simulink model "VACModel"  (Simulink 8.3)
settings: Solver=ode1  SolverMode=MultiTasking  StartTime=0.0  StopTime=24  FixedStep=Ts_base  MaxStep=Ts_base  MinStep=1e-6  RelTol=1e-6
PreLoadFcn:
  | initModel
StopFcn:
  | overview
undefined symbols (not defined in the file): automatic, controller_sampling_frequency, Fixed, gcr, MVs, PI, signal, transmitter_deadtime, transmitter_sampling_frequency, Ts_save, y_ss
libraries: VAlib x96
(part 15 of 18)

== system VACModel/VA Plant/xmeas atk block/xmeas3 attack controller/Attack Type Controller ==
  note: 1) Only subsystems can be added as variant choices at this level
      | 2) Blocks cannot be connected at this level as connectivity is
      | automatically determined at simulation, based on the active variant
  normal : Inport
  faked : Inport  Port=2
  interval forward controller : Subsystem  VariantControl=interval_forward_controller
      mask Display:
      | disp('IFC')
      | port_label('input', 1, 'normal in')
      | port_label('input', 2, 'faked in')
      | port_label('output', 1, 'out')
  normal forward controller : Subsystem  VariantControl=normal_forward_controller
      mask Display:
      | disp('NFC')
      | port_label('input', 1, 'normal in')
      | port_label('input', 2, 'faked in')
      | port_label('output', 1, 'out')
  periodical forward controller : Subsystem  VariantControl=periodical_forward_controller
      mask Display:
      | disp('PFC')
      | port_label('input', 1, 'normal in')
      | port_label('input', 2, 'faked in')
      | port_label('output', 1, 'out')
  step forward controller : Subsystem  VariantControl=step_forward_controller
      mask Display:
      | disp('SFC')
      | port_label('input', 1, 'normal in')
      | port_label('input', 2, 'faked in')
      | port_label('output', 1, 'out')
  output : Outport

== system VACModel/VA Plant/xmeas atk block/xmeas30 attack controller/Attack Type Controller ==
  note: 1) Only subsystems can be added as variant choices at this level
      | 2) Blocks cannot be connected at this level as connectivity is
      | automatically determined at simulation, based on the active variant
  normal : Inport
  faked : Inport  Port=2
  interval forward controller : Subsystem  VariantControl=interval_forward_controller
      mask Display:
      | disp('IFC')
      | port_label('input', 1, 'normal in')
      | port_label('input', 2, 'faked in')
      | port_label('output', 1, 'out')
  normal forward controller : Subsystem  VariantControl=normal_forward_controller
      mask Display:
      | disp('NFC')
      | port_label('input', 1, 'normal in')
      | port_label('input', 2, 'faked in')
      | port_label('output', 1, 'out')
  periodical forward controller : Subsystem  VariantControl=periodical_forward_controller
      mask Display:
      | disp('PFC')
      | port_label('input', 1, 'normal in')
      | port_label('input', 2, 'faked in')
      | port_label('output', 1, 'out')
  step forward controller : Subsystem  VariantControl=step_forward_controller
      mask Display:
      | disp('SFC')
      | port_label('input', 1, 'normal in')
      | port_label('input', 2, 'faked in')
      | port_label('output', 1, 'out')
  output : Outport

== system VACModel/VA Plant/xmeas atk block/xmeas31 attack controller/Attack Type Controller ==
  note: 1) Only subsystems can be added as variant choices at this level
      | 2) Blocks cannot be connected at this level as connectivity is
      | automatically determined at simulation, based on the active variant
  normal : Inport
  faked : Inport  Port=2
  interval forward controller : Subsystem  VariantControl=interval_forward_controller
      mask Display:
      | disp('IFC')
      | port_label('input', 1, 'normal in')
      | port_label('input', 2, 'faked in')
      | port_label('output', 1, 'out')
  normal forward controller : Subsystem  VariantControl=normal_forward_controller
      mask Display:
      | disp('NFC')
      | port_label('input', 1, 'normal in')
      | port_label('input', 2, 'faked in')
      | port_label('output', 1, 'out')
  periodical forward controller : Subsystem  VariantControl=periodical_forward_controller
      mask Display:
      | disp('PFC')
      | port_label('input', 1, 'normal in')
      | port_label('input', 2, 'faked in')
      | port_label('output', 1, 'out')
  step forward controller : Subsystem  VariantControl=step_forward_controller
      mask Display:
      | disp('SFC')
      | port_label('input', 1, 'normal in')
      | port_label('input', 2, 'faked in')
      | port_label('output', 1, 'out')
  output : Outport

== system VACModel/VA Plant/xmeas atk block/xmeas32 attack controller/Attack Type Controller ==
  note: 1) Only subsystems can be added as variant choices at this level
      | 2) Blocks cannot be connected at this level as connectivity is
      | automatically determined at simulation, based on the active variant
  normal : Inport
  faked : Inport  Port=2
  interval forward controller : Subsystem  VariantControl=interval_forward_controller
      mask Display:
      | disp('IFC')
      | port_label('input', 1, 'normal in')
      | port_label('input', 2, 'faked in')
      | port_label('output', 1, 'out')
  normal forward controller : Subsystem  VariantControl=normal_forward_controller
      mask Display:
      | disp('NFC')
      | port_label('input', 1, 'normal in')
      | port_label('input', 2, 'faked in')
      | port_label('output', 1, 'out')
  periodical forward controller : Subsystem  VariantControl=periodical_forward_controller
      mask Display:
      | disp('PFC')
      | port_label('input', 1, 'normal in')
      | port_label('input', 2, 'faked in')
      | port_label('output', 1, 'out')
  step forward controller : Subsystem  VariantControl=step_forward_controller
      mask Display:
      | disp('SFC')
      | port_label('input', 1, 'normal in')
      | port_label('input', 2, 'faked in')
      | port_label('output', 1, 'out')
  output : Outport

== system VACModel/VA Plant/xmeas atk block/xmeas33 attack controller/Attack Type Controller ==
  note: 1) Only subsystems can be added as variant choices at this level
      | 2) Blocks cannot be connected at this level as connectivity is
      | automatically determined at simulation, based on the active variant
  normal : Inport
  faked : Inport  Port=2
  interval forward controller : Subsystem  VariantControl=interval_forward_controller
      mask Display:
      | disp('IFC')
      | port_label('input', 1, 'normal in')
      | port_label('input', 2, 'faked in')
      | port_label('output', 1, 'out')
  normal forward controller : Subsystem  VariantControl=normal_forward_controller
      mask Display:
      | disp('NFC')
      | port_label('input', 1, 'normal in')
      | port_label('input', 2, 'faked in')
      | port_label('output', 1, 'out')
  periodical forward controller : Subsystem  VariantControl=periodical_forward_controller
      mask Display:
      | disp('PFC')
      | port_label('input', 1, 'normal in')
      | port_label('input', 2, 'faked in')
      | port_label('output', 1, 'out')
  step forward controller : Subsystem  VariantControl=step_forward_controller
      mask Display:
      | disp('SFC')
      | port_label('input', 1, 'normal in')
      | port_label('input', 2, 'faked in')
      | port_label('output', 1, 'out')
  output : Outport

== system VACModel/VA Plant/xmeas atk block/xmeas34 attack controller/Attack Type Controller ==
  note: 1) Only subsystems can be added as variant choices at this level
      | 2) Blocks cannot be connected at this level as connectivity is
      | automatically determined at simulation, based on the active variant
  normal : Inport
  faked : Inport  Port=2
  interval forward controller : Subsystem  VariantControl=interval_forward_controller
      mask Display:
      | disp('IFC')
      | port_label('input', 1, 'normal in')
      | port_label('input', 2, 'faked in')
      | port_label('output', 1, 'out')
  normal forward controller : Subsystem  VariantControl=normal_forward_controller
      mask Display:
      | disp('NFC')
      | port_label('input', 1, 'normal in')
      | port_label('input', 2, 'faked in')
      | port_label('output', 1, 'out')
  periodical forward controller : Subsystem  VariantControl=periodical_forward_controller
      mask Display:
      | disp('PFC')
      | port_label('input', 1, 'normal in')
      | port_label('input', 2, 'faked in')
      | port_label('output', 1, 'out')
  step forward controller : Subsystem  VariantControl=step_forward_controller
      mask Display:
      | disp('SFC')
      | port_label('input', 1, 'normal in')
      | port_label('input', 2, 'faked in')
      | port_label('output', 1, 'out')
  output : Outport

== system VACModel/VA Plant/xmeas atk block/xmeas35 attack controller/Attack Type Controller ==
  note: 1) Only subsystems can be added as variant choices at this level
      | 2) Blocks cannot be connected at this level as connectivity is
      | automatically determined at simulation, based on the active variant
  normal : Inport
  faked : Inport  Port=2
  interval forward controller : Subsystem  VariantControl=interval_forward_controller
      mask Display:
      | disp('IFC')
      | port_label('input', 1, 'normal in')
      | port_label('input', 2, 'faked in')
      | port_label('output', 1, 'out')
  normal forward controller : Subsystem  VariantControl=normal_forward_controller
      mask Display:
      | disp('NFC')
      | port_label('input', 1, 'normal in')
      | port_label('input', 2, 'faked in')
      | port_label('output', 1, 'out')
  periodical forward controller : Subsystem  VariantControl=periodical_forward_controller
      mask Display:
      | disp('PFC')
      | port_label('input', 1, 'normal in')
      | port_label('input', 2, 'faked in')
      | port_label('output', 1, 'out')
  step forward controller : Subsystem  VariantControl=step_forward_controller
      mask Display:
      | disp('SFC')
      | port_label('input', 1, 'normal in')
      | port_label('input', 2, 'faked in')
      | port_label('output', 1, 'out')
  output : Outport

== system VACModel/VA Plant/xmeas atk block/xmeas36 attack controller/Attack Type Controller ==
  note: 1) Only subsystems can be added as variant choices at this level
      | 2) Blocks cannot be connected at this level as connectivity is
      | automatically determined at simulation, based on the active variant
  normal : Inport
  faked : Inport  Port=2
  interval forward controller : Subsystem  VariantControl=interval_forward_controller
      mask Display:
      | disp('IFC')
      | port_label('input', 1, 'normal in')
      | port_label('input', 2, 'faked in')
      | port_label('output', 1, 'out')
  normal forward controller : Subsystem  VariantControl=normal_forward_controller
      mask Display:
      | disp('NFC')
      | port_label('input', 1, 'normal in')
      | port_label('input', 2, 'faked in')
      | port_label('output', 1, 'out')
  periodical forward controller : Subsystem  VariantControl=periodical_forward_controller
      mask Display:
      | disp('PFC')
      | port_label('input', 1, 'normal in')
      | port_label('input', 2, 'faked in')
      | port_label('output', 1, 'out')
  step forward controller : Subsystem  VariantControl=step_forward_controller
      mask Display:
      | disp('SFC')
      | port_label('input', 1, 'normal in')
      | port_label('input', 2, 'faked in')
      | port_label('output', 1, 'out')
  output : Outport

== system VACModel/VA Plant/xmeas atk block/xmeas37 attack controller/Attack Type Controller ==
  note: 1) Only subsystems can be added as variant choices at this level
      | 2) Blocks cannot be connected at this level as connectivity is
      | automatically determined at simulation, based on the active variant
  normal : Inport
  faked : Inport  Port=2
  interval forward controller : Subsystem  VariantControl=interval_forward_controller
      mask Display:
      | disp('IFC')
      | port_label('input', 1, 'normal in')
      | port_label('input', 2, 'faked in')
      | port_label('output', 1, 'out')
  normal forward controller : Subsystem  VariantControl=normal_forward_controller
      mask Display:
      | disp('NFC')
      | port_label('input', 1, 'normal in')
      | port_label('input', 2, 'faked in')
      | port_label('output', 1, 'out')
  periodical forward controller : Subsystem  VariantControl=periodical_forward_controller
      mask Display:
      | disp('PFC')
      | port_label('input', 1, 'normal in')
      | port_label('input', 2, 'faked in')
      | port_label('output', 1, 'out')
  step forward controller : Subsystem  VariantControl=step_forward_controller
      mask Display:
      | disp('SFC')
      | port_label('input', 1, 'normal in')
      | port_label('input', 2, 'faked in')
      | port_label('output', 1, 'out')
  output : Outport

== system VACModel/VA Plant/xmeas atk block/xmeas38 attack controller/Attack Type Controller ==
  note: 1) Only subsystems can be added as variant choices at this level
      | 2) Blocks cannot be connected at this level as connectivity is
      | automatically determined at simulation, based on the active variant
  normal : Inport
  faked : Inport  Port=2
  interval forward controller : Subsystem  VariantControl=interval_forward_controller
      mask Display:
      | disp('IFC')
      | port_label('input', 1, 'normal in')
      | port_label('input', 2, 'faked in')
      | port_label('output', 1, 'out')
  normal forward controller : Subsystem  VariantControl=normal_forward_controller
      mask Display:
      | disp('NFC')
      | port_label('input', 1, 'normal in')
      | port_label('input', 2, 'faked in')
      | port_label('output', 1, 'out')
  periodical forward controller : Subsystem  VariantControl=periodical_forward_controller
      mask Display:
      | disp('PFC')
      | port_label('input', 1, 'normal in')
      | port_label('input', 2, 'faked in')
      | port_label('output', 1, 'out')
  step forward controller : Subsystem  VariantControl=step_forward_controller
      mask Display:
      | disp('SFC')
      | port_label('input', 1, 'normal in')
      | port_label('input', 2, 'faked in')
      | port_label('output', 1, 'out')
  output : Outport

== system VACModel/VA Plant/xmeas atk block/xmeas39 attack controller/Attack Type Controller ==
  note: 1) Only subsystems can be added as variant choices at this level
      | 2) Blocks cannot be connected at this level as connectivity is
      | automatically determined at simulation, based on the active variant
  normal : Inport
  faked : Inport  Port=2
  interval forward controller : Subsystem  VariantControl=interval_forward_controller
      mask Display:
      | disp('IFC')
      | port_label('input', 1, 'normal in')
      | port_label('input', 2, 'faked in')
      | port_label('output', 1, 'out')
  normal forward controller : Subsystem  VariantControl=normal_forward_controller
      mask Display:
      | disp('NFC')
      | port_label('input', 1, 'normal in')
      | port_label('input', 2, 'faked in')
      | port_label('output', 1, 'out')
  periodical forward controller : Subsystem  VariantControl=periodical_forward_controller
      mask Display:
      | disp('PFC')
      | port_label('input', 1, 'normal in')
      | port_label('input', 2, 'faked in')
      | port_label('output', 1, 'out')
  step forward controller : Subsystem  VariantControl=step_forward_controller
      mask Display:
      | disp('SFC')
      | port_label('input', 1, 'normal in')
      | port_label('input', 2, 'faked in')
      | port_label('output', 1, 'out')
  output : Outport

== system VACModel/VA Plant/xmeas atk block/xmeas4 attack controller/Attack Type Controller ==
  note: 1) Only subsystems can be added as variant choices at this level
      | 2) Blocks cannot be connected at this level as connectivity is
      | automatically determined at simulation, based on the active variant
  normal : Inport
  faked : Inport  Port=2
  interval forward controller : Subsystem  VariantControl=interval_forward_controller
      mask Display:
      | disp('IFC')
      | port_label('input', 1, 'normal in')
      | port_label('input', 2, 'faked in')
      | port_label('output', 1, 'out')
  normal forward controller : Subsystem  VariantControl=normal_forward_controller
      mask Display:
      | disp('NFC')
      | port_label('input', 1, 'normal in')
      | port_label('input', 2, 'faked in')
      | port_label('output', 1, 'out')
  periodical forward controller : Subsystem  VariantControl=periodical_forward_controller
      mask Display:
      | disp('PFC')
      | port_label('input', 1, 'normal in')
      | port_label('input', 2, 'faked in')
      | port_label('output', 1, 'out')
  step forward controller : Subsystem  VariantControl=step_forward_controller
      mask Display:
      | disp('SFC')
      | port_label('input', 1, 'normal in')
      | port_label('input', 2, 'faked in')
      | port_label('output', 1, 'out')
  output : Outport

== system VACModel/VA Plant/xmeas atk block/xmeas40 attack controller/Attack Type Controller ==
  note: 1) Only subsystems can be added as variant choices at this level
      | 2) Blocks cannot be connected at this level as connectivity is
      | automatically determined at simulation, based on the active variant
  normal : Inport
  faked : Inport  Port=2
  interval forward controller : Subsystem  VariantControl=interval_forward_controller
      mask Display:
      | disp('IFC')
      | port_label('input', 1, 'normal in')
      | port_label('input', 2, 'faked in')
      | port_label('output', 1, 'out')
  normal forward controller : Subsystem  VariantControl=normal_forward_controller
      mask Display:
      | disp('NFC')
      | port_label('input', 1, 'normal in')
      | port_label('input', 2, 'faked in')
      | port_label('output', 1, 'out')
  periodical forward controller : Subsystem  VariantControl=periodical_forward_controller
      mask Display:
      | disp('PFC')
      | port_label('input', 1, 'normal in')
      | port_label('input', 2, 'faked in')
      | port_label('output', 1, 'out')
  step forward controller : Subsystem  VariantControl=step_forward_controller
      mask Display:
      | disp('SFC')
      | port_label('input', 1, 'normal in')
      | port_label('input', 2, 'faked in')
      | port_label('output', 1, 'out')
  output : Outport

== system VACModel/VA Plant/xmeas atk block/xmeas41 attack controller/Attack Type Controller ==
  note: 1) Only subsystems can be added as variant choices at this level
      | 2) Blocks cannot be connected at this level as connectivity is
      | automatically determined at simulation, based on the active variant
  normal : Inport
  faked : Inport  Port=2
  interval forward controller : Subsystem  VariantControl=interval_forward_controller
      mask Display:
      | disp('IFC')
      | port_label('input', 1, 'normal in')
      | port_label('input', 2, 'faked in')
      | port_label('output', 1, 'out')
  normal forward controller : Subsystem  VariantControl=normal_forward_controller
      mask Display:
      | disp('NFC')
      | port_label('input', 1, 'normal in')
      | port_label('input', 2, 'faked in')
      | port_label('output', 1, 'out')
  periodical forward controller : Subsystem  VariantControl=periodical_forward_controller
      mask Display:
      | disp('PFC')
      | port_label('input', 1, 'normal in')
      | port_label('input', 2, 'faked in')
      | port_label('output', 1, 'out')
  step forward controller : Subsystem  VariantControl=step_forward_controller
      mask Display:
      | disp('SFC')
      | port_label('input', 1, 'normal in')
      | port_label('input', 2, 'faked in')
      | port_label('output', 1, 'out')
  output : Outport

== system VACModel/VA Plant/xmeas atk block/xmeas42 attack controller/Attack Type Controller ==
  note: 1) Only subsystems can be added as variant choices at this level
      | 2) Blocks cannot be connected at this level as connectivity is
      | automatically determined at simulation, based on the active variant
  normal : Inport
  faked : Inport  Port=2
  interval forward controller : Subsystem  VariantControl=interval_forward_controller
      mask Display:
      | disp('IFC')
      | port_label('input', 1, 'normal in')
      | port_label('input', 2, 'faked in')
      | port_label('output', 1, 'out')
  normal forward controller : Subsystem  VariantControl=normal_forward_controller
      mask Display:
      | disp('NFC')
      | port_label('input', 1, 'normal in')
      | port_label('input', 2, 'faked in')
      | port_label('output', 1, 'out')
  periodical forward controller : Subsystem  VariantControl=periodical_forward_controller
      mask Display:
      | disp('PFC')
      | port_label('input', 1, 'normal in')
      | port_label('input', 2, 'faked in')
      | port_label('output', 1, 'out')
  step forward controller : Subsystem  VariantControl=step_forward_controller
      mask Display:
      | disp('SFC')
      | port_label('input', 1, 'normal in')
      | port_label('input', 2, 'faked in')
      | port_label('output', 1, 'out')
  output : Outport

== system VACModel/VA Plant/xmeas atk block/xmeas43 attack controller/Attack Type Controller ==
  note: 1) Only subsystems can be added as variant choices at this level
      | 2) Blocks cannot be connected at this level as connectivity is
      | automatically determined at simulation, based on the active variant
  normal : Inport
  faked : Inport  Port=2
  interval forward controller : Subsystem  VariantControl=interval_forward_controller
      mask Display:
      | disp('IFC')
      | port_label('input', 1, 'normal in')
      | port_label('input', 2, 'faked in')
      | port_label('output', 1, 'out')
  normal forward controller : Subsystem  VariantControl=normal_forward_controller
      mask Display:
      | disp('NFC')
      | port_label('input', 1, 'normal in')
      | port_label('input', 2, 'faked in')
      | port_label('output', 1, 'out')
  periodical forward controller : Subsystem  VariantControl=periodical_forward_controller
      mask Display:
      | disp('PFC')
      | port_label('input', 1, 'normal in')
      | port_label('input', 2, 'faked in')
      | port_label('output', 1, 'out')
  step forward controller : Subsystem  VariantControl=step_forward_controller
      mask Display:
      | disp('SFC')
      | port_label('input', 1, 'normal in')
      | port_label('input', 2, 'faked in')
      | port_label('output', 1, 'out')
  output : Outport

== system VACModel/VA Plant/xmeas atk block/xmeas5 attack controller/Attack Type Controller ==
  note: 1) Only subsystems can be added as variant choices at this level
      | 2) Blocks cannot be connected at this level as connectivity is
      | automatically determined at simulation, based on the active variant
  normal : Inport
  faked : Inport  Port=2
  interval forward controller : Subsystem  VariantControl=interval_forward_controller
      mask Display:
      | disp('IFC')
      | port_label('input', 1, 'normal in')
      | port_label('input', 2, 'faked in')
      | port_label('output', 1, 'out')
  normal forward controller : Subsystem  VariantControl=normal_forward_controller
      mask Display:
      | disp('NFC')
      | port_label('input', 1, 'normal in')
      | port_label('input', 2, 'faked in')
      | port_label('output', 1, 'out')
  periodical forward controller : Subsystem  VariantControl=periodical_forward_controller
      mask Display:
      | disp('PFC')
      | port_label('input', 1, 'normal in')
      | port_label('input', 2, 'faked in')
      | port_label('output', 1, 'out')
  step forward controller : Subsystem  VariantControl=step_forward_controller
      mask Display:
      | disp('SFC')
      | port_label('input', 1, 'normal in')
      | port_label('input', 2, 'faked in')
      | port_label('output', 1, 'out')
  output : Outport

== system VACModel/VA Plant/xmeas atk block/xmeas6 attack controller/Attack Type Controller ==
  note: 1) Only subsystems can be added as variant choices at this level
      | 2) Blocks cannot be connected at this level as connectivity is
      | automatically determined at simulation, based on the active variant
  normal : Inport
  faked : Inport  Port=2
  interval forward controller : Subsystem  VariantControl=interval_forward_controller
      mask Display:
      | disp('IFC')
      | port_label('input', 1, 'normal in')
      | port_label('input', 2, 'faked in')
      | port_label('output', 1, 'out')
  normal forward controller : Subsystem  VariantControl=normal_forward_controller
      mask Display:
      | disp('NFC')
      | port_label('input', 1, 'normal in')
      | port_label('input', 2, 'faked in')
      | port_label('output', 1, 'out')
  periodical forward controller : Subsystem  VariantControl=periodical_forward_controller
      mask Display:
      | disp('PFC')
      | port_label('input', 1, 'normal in')
      | port_label('input', 2, 'faked in')
      | port_label('output', 1, 'out')
  step forward controller : Subsystem  VariantControl=step_forward_controller
      mask Display:
      | disp('SFC')
      | port_label('input', 1, 'normal in')
      | port_label('input', 2, 'faked in')
      | port_label('output', 1, 'out')
  output : Outport

== system VACModel/VA Plant/xmeas atk block/xmeas7 attack controller/Attack Type Controller ==
  note: 1) Only subsystems can be added as variant choices at this level
      | 2) Blocks cannot be connected at this level as connectivity is
      | automatically determined at simulation, based on the active variant
  normal : Inport
  faked : Inport  Port=2
  interval forward controller : Subsystem  VariantControl=interval_forward_controller
      mask Display:
      | disp('IFC')
      | port_label('input', 1, 'normal in')
      | port_label('input', 2, 'faked in')
      | port_label('output', 1, 'out')
  normal forward controller : Subsystem  VariantControl=normal_forward_controller
      mask Display:
      | disp('NFC')
      | port_label('input', 1, 'normal in')
      | port_label('input', 2, 'faked in')
      | port_label('output', 1, 'out')
  periodical forward controller : Subsystem  VariantControl=periodical_forward_controller
      mask Display:
      | disp('PFC')
      | port_label('input', 1, 'normal in')
      | port_label('input', 2, 'faked in')
      | port_label('output', 1, 'out')
  step forward controller : Subsystem  VariantControl=step_forward_controller
      mask Display:
      | disp('SFC')
      | port_label('input', 1, 'normal in')
      | port_label('input', 2, 'faked in')
      | port_label('output', 1, 'out')
  output : Outport

== system VACModel/VA Plant/xmeas atk block/xmeas8 attack controller/Attack Type Controller ==
  note: 1) Only subsystems can be added as variant choices at this level
      | 2) Blocks cannot be connected at this level as connectivity is
      | automatically determined at simulation, based on the active variant
  normal : Inport
  faked : Inport  Port=2
  interval forward controller : Subsystem  VariantControl=interval_forward_controller
      mask Display:
      | disp('IFC')
      | port_label('input', 1, 'normal in')
      | port_label('input', 2, 'faked in')
      | port_label('output', 1, 'out')
  normal forward controller : Subsystem  VariantControl=normal_forward_controller
      mask Display:
      | disp('NFC')
      | port_label('input', 1, 'normal in')
      | port_label('input', 2, 'faked in')
      | port_label('output', 1, 'out')
  periodical forward controller : Subsystem  VariantControl=periodical_forward_controller
      mask Display:
      | disp('PFC')
      | port_label('input', 1, 'normal in')
      | port_label('input', 2, 'faked in')
      | port_label('output', 1, 'out')
  step forward controller : Subsystem  VariantControl=step_forward_controller
      mask Display:
      | disp('SFC')
      | port_label('input', 1, 'normal in')
      | port_label('input', 2, 'faked in')
      | port_label('output', 1, 'out')
  output : Outport

== system VACModel/VA Plant/xmeas atk block/xmeas9 attack controller/Attack Type Controller ==
  note: 1) Only subsystems can be added as variant choices at this level
      | 2) Blocks cannot be connected at this level as connectivity is
      | automatically determined at simulation, based on the active variant
  normal : Inport
  faked : Inport  Port=2
  interval forward controller : Subsystem  VariantControl=interval_forward_controller
      mask Display:
      | disp('IFC')
      | port_label('input', 1, 'normal in')
      | port_label('input', 2, 'faked in')
      | port_label('output', 1, 'out')
  normal forward controller : Subsystem  VariantControl=normal_forward_controller
      mask Display:
      | disp('NFC')
      | port_label('input', 1, 'normal in')
      | port_label('input', 2, 'faked in')
      | port_label('output', 1, 'out')
  periodical forward controller : Subsystem  VariantControl=periodical_forward_controller
      mask Display:
      | disp('PFC')
      | port_label('input', 1, 'normal in')
      | port_label('input', 2, 'faked in')
      | port_label('output', 1, 'out')
  step forward controller : Subsystem  VariantControl=step_forward_controller
      mask Display:
      | disp('SFC')
      | port_label('input', 1, 'normal in')
      | port_label('input', 2, 'faked in')
      | port_label('output', 1, 'out')
  output : Outport

== system VACModel/VA Plant/xmv atk block/xmv1 attack controller/Attack Type Controller ==
  note: 1) Only subsystems can be added as variant choices at this level
      | 2) Blocks cannot be connected at this level as connectivity is
      | automatically determined at simulation, based on the active variant
  normal : Inport
  faked : Inport  Port=2
  interval forward controller : Subsystem  VariantControl=interval_forward_controller
      mask Display:
      | disp('IFC')
      | port_label('input', 1, 'normal in')
      | port_label('input', 2, 'faked in')
      | port_label('output', 1, 'out')
  normal forward controller : Subsystem  VariantControl=normal_forward_controller
      mask Display:
      | disp('NFC')
      | port_label('input', 1, 'normal in')
      | port_label('input', 2, 'faked in')
      | port_label('output', 1, 'out')
  periodical forward controller : Subsystem  VariantControl=periodical_forward_controller
      mask Display:
      | disp('PFC')
      | port_label('input', 1, 'normal in')
      | port_label('input', 2, 'faked in')
      | port_label('output', 1, 'out')
  step forward controller : Subsystem  VariantControl=step_forward_controller
      mask Display:
      | disp('SFC')
      | port_label('input', 1, 'normal in')
      | port_label('input', 2, 'faked in')
      | port_label('output', 1, 'out')
  output : Outport

== system VACModel/VA Plant/xmv atk block/xmv10 attack controller/Attack Type Controller ==
  note: 1) Only subsystems can be added as variant choices at this level
      | 2) Blocks cannot be connected at this level as connectivity is
      | automatically determined at simulation, based on the active variant
  normal : Inport
  faked : Inport  Port=2
  interval forward controller : Subsystem  VariantControl=interval_forward_controller
      mask Display:
      | disp('IFC')
      | port_label('input', 1, 'normal in')
      | port_label('input', 2, 'faked in')
      | port_label('output', 1, 'out')
  normal forward controller : Subsystem  VariantControl=normal_forward_controller
      mask Display:
      | disp('NFC')
      | port_label('input', 1, 'normal in')
      | port_label('input', 2, 'faked in')
      | port_label('output', 1, 'out')
  periodical forward controller : Subsystem  VariantControl=periodical_forward_controller
      mask Display:
      | disp('PFC')
      | port_label('input', 1, 'normal in')
      | port_label('input', 2, 'faked in')
      | port_label('output', 1, 'out')
  step forward controller : Subsystem  VariantControl=step_forward_controller
      mask Display:
      | disp('SFC')
      | port_label('input', 1, 'normal in')
      | port_label('input', 2, 'faked in')
      | port_label('output', 1, 'out')
  output : Outport

== system VACModel/VA Plant/xmv atk block/xmv11 attack controller/Attack Type Controller ==
  note: 1) Only subsystems can be added as variant choices at this level
      | 2) Blocks cannot be connected at this level as connectivity is
      | automatically determined at simulation, based on the active variant
  normal : Inport
  faked : Inport  Port=2
  interval forward controller : Subsystem  VariantControl=interval_forward_controller
      mask Display:
      | disp('IFC')
      | port_label('input', 1, 'normal in')
      | port_label('input', 2, 'faked in')
      | port_label('output', 1, 'out')
  normal forward controller : Subsystem  VariantControl=normal_forward_controller
      mask Display:
      | disp('NFC')
      | port_label('input', 1, 'normal in')
      | port_label('input', 2, 'faked in')
      | port_label('output', 1, 'out')
  periodical forward controller : Subsystem  VariantControl=periodical_forward_controller
      mask Display:
      | disp('PFC')
      | port_label('input', 1, 'normal in')
      | port_label('input', 2, 'faked in')
      | port_label('output', 1, 'out')
  step forward controller : Subsystem  VariantControl=step_forward_controller
      mask Display:
      | disp('SFC')
      | port_label('input', 1, 'normal in')
      | port_label('input', 2, 'faked in')
      | port_label('output', 1, 'out')
  output : Outport

== system VACModel/VA Plant/xmv atk block/xmv12 attack controller/Attack Type Controller ==
  note: 1) Only subsystems can be added as variant choices at this level
      | 2) Blocks cannot be connected at this level as connectivity is
      | automatically determined at simulation, based on the active variant
  normal : Inport
  faked : Inport  Port=2
  interval forward controller : Subsystem  VariantControl=interval_forward_controller
      mask Display:
      | disp('IFC')
      | port_label('input', 1, 'normal in')
      | port_label('input', 2, 'faked in')
      | port_label('output', 1, 'out')
  normal forward controller : Subsystem  VariantControl=normal_forward_controller
      mask Display:
      | disp('NFC')
      | port_label('input', 1, 'normal in')
      | port_label('input', 2, 'faked in')
      | port_label('output', 1, 'out')
  periodical forward controller : Subsystem  VariantControl=periodical_forward_controller
      mask Display:
      | disp('PFC')
      | port_label('input', 1, 'normal in')
      | port_label('input', 2, 'faked in')
      | port_label('output', 1, 'out')
  step forward controller : Subsystem  VariantControl=step_forward_controller
      mask Display:
      | disp('SFC')
      | port_label('input', 1, 'normal in')
      | port_label('input', 2, 'faked in')
      | port_label('output', 1, 'out')
  output : Outport

== system VACModel/VA Plant/xmv atk block/xmv13 attack controller/Attack Type Controller ==
  note: 1) Only subsystems can be added as variant choices at this level
      | 2) Blocks cannot be connected at this level as connectivity is
      | automatically determined at simulation, based on the active variant
  normal : Inport
  faked : Inport  Port=2
  interval forward controller : Subsystem  VariantControl=interval_forward_controller
      mask Display:
      | disp('IFC')
      | port_label('input', 1, 'normal in')
      | port_label('input', 2, 'faked in')
      | port_label('output', 1, 'out')
  normal forward controller : Subsystem  VariantControl=normal_forward_controller
      mask Display:
      | disp('NFC')
      | port_label('input', 1, 'normal in')
      | port_label('input', 2, 'faked in')
      | port_label('output', 1, 'out')
  periodical forward controller : Subsystem  VariantControl=periodical_forward_controller
      mask Display:
      | disp('PFC')
      | port_label('input', 1, 'normal in')
      | port_label('input', 2, 'faked in')
      | port_label('output', 1, 'out')
  step forward controller : Subsystem  VariantControl=step_forward_controller
      mask Display:
      | disp('SFC')
      | port_label('input', 1, 'normal in')
      | port_label('input', 2, 'faked in')
      | port_label('output', 1, 'out')
  output : Outport

== system VACModel/VA Plant/xmv atk block/xmv14 attack controller/Attack Type Controller ==
  note: 1) Only subsystems can be added as variant choices at this level
      | 2) Blocks cannot be connected at this level as connectivity is
      | automatically determined at simulation, based on the active variant
  normal : Inport
  faked : Inport  Port=2
  interval forward controller : Subsystem  VariantControl=interval_forward_controller
      mask Display:
      | disp('IFC')
      | port_label('input', 1, 'normal in')
      | port_label('input', 2, 'faked in')
      | port_label('output', 1, 'out')
  normal forward controller : Subsystem  VariantControl=normal_forward_controller
      mask Display:
      | disp('NFC')
      | port_label('input', 1, 'normal in')
      | port_label('input', 2, 'faked in')
      | port_label('output', 1, 'out')
  periodical forward controller : Subsystem  VariantControl=periodical_forward_controller
      mask Display:
      | disp('PFC')
      | port_label('input', 1, 'normal in')
      | port_label('input', 2, 'faked in')
      | port_label('output', 1, 'out')
  step forward controller : Subsystem  VariantControl=step_forward_controller
      mask Display:
      | disp('SFC')
      | port_label('input', 1, 'normal in')
      | port_label('input', 2, 'faked in')
      | port_label('output', 1, 'out')
  output : Outport

== system VACModel/VA Plant/xmv atk block/xmv15 attack controller/Attack Type Controller ==
  note: 1) Only subsystems can be added as variant choices at this level
      | 2) Blocks cannot be connected at this level as connectivity is
      | automatically determined at simulation, based on the active variant
  normal : Inport
  faked : Inport  Port=2
  interval forward controller : Subsystem  VariantControl=interval_forward_controller
      mask Display:
      | disp('IFC')
      | port_label('input', 1, 'normal in')
      | port_label('input', 2, 'faked in')
      | port_label('output', 1, 'out')
  normal forward controller : Subsystem  VariantControl=normal_forward_controller
      mask Display:
      | disp('NFC')
      | port_label('input', 1, 'normal in')
      | port_label('input', 2, 'faked in')
      | port_label('output', 1, 'out')
  periodical forward controller : Subsystem  VariantControl=periodical_forward_controller
      mask Display:
      | disp('PFC')
      | port_label('input', 1, 'normal in')
      | port_label('input', 2, 'faked in')
      | port_label('output', 1, 'out')
  step forward controller : Subsystem  VariantControl=step_forward_controller
      mask Display:
      | disp('SFC')
      | port_label('input', 1, 'normal in')
      | port_label('input', 2, 'faked in')
      | port_label('output', 1, 'out')
  output : Outport

== system VACModel/VA Plant/xmv atk block/xmv16 attack controller/Attack Type Controller ==
  note: 1) Only subsystems can be added as variant choices at this level
      | 2) Blocks cannot be connected at this level as connectivity is
      | automatically determined at simulation, based on the active variant
  normal : Inport
  faked : Inport  Port=2
  interval forward controller : Subsystem  VariantControl=interval_forward_controller
      mask Display:
      | disp('IFC')
      | port_label('input', 1, 'normal in')
      | port_label('input', 2, 'faked in')
      | port_label('output', 1, 'out')
  normal forward controller : Subsystem  VariantControl=normal_forward_controller
      mask Display:
      | disp('NFC')
      | port_label('input', 1, 'normal in')
      | port_label('input', 2, 'faked in')
      | port_label('output', 1, 'out')
  periodical forward controller : Subsystem  VariantControl=periodical_forward_controller
      mask Display:
      | disp('PFC')
      | port_label('input', 1, 'normal in')
      | port_label('input', 2, 'faked in')
      | port_label('output', 1, 'out')
  step forward controller : Subsystem  VariantControl=step_forward_controller
      mask Display:
      | disp('SFC')
      | port_label('input', 1, 'normal in')
      | port_label('input', 2, 'faked in')
      | port_label('output', 1, 'out')
  output : Outport

== system VACModel/VA Plant/xmv atk block/xmv17 attack controller/Attack Type Controller ==
  note: 1) Only subsystems can be added as variant choices at this level
      | 2) Blocks cannot be connected at this level as connectivity is
      | automatically determined at simulation, based on the active variant
  normal : Inport
  faked : Inport  Port=2
  interval forward controller : Subsystem  VariantControl=interval_forward_controller
      mask Display:
      | disp('IFC')
      | port_label('input', 1, 'normal in')
      | port_label('input', 2, 'faked in')
      | port_label('output', 1, 'out')
  normal forward controller : Subsystem  VariantControl=normal_forward_controller
      mask Display:
      | disp('NFC')
      | port_label('input', 1, 'normal in')
      | port_label('input', 2, 'faked in')
      | port_label('output', 1, 'out')
  periodical forward controller : Subsystem  VariantControl=periodical_forward_controller
      mask Display:
      | disp('PFC')
      | port_label('input', 1, 'normal in')
      | port_label('input', 2, 'faked in')
      | port_label('output', 1, 'out')
  step forward controller : Subsystem  VariantControl=step_forward_controller
      mask Display:
      | disp('SFC')
      | port_label('input', 1, 'normal in')
      | port_label('input', 2, 'faked in')
      | port_label('output', 1, 'out')
  output : Outport

== system VACModel/VA Plant/xmv atk block/xmv18 attack controller/Attack Type Controller ==
  note: 1) Only subsystems can be added as variant choices at this level
      | 2) Blocks cannot be connected at this level as connectivity is
      | automatically determined at simulation, based on the active variant
  normal : Inport
  faked : Inport  Port=2
  interval forward controller : Subsystem  VariantControl=interval_forward_controller
      mask Display:
      | disp('IFC')
      | port_label('input', 1, 'normal in')
      | port_label('input', 2, 'faked in')
      | port_label('output', 1, 'out')
  normal forward controller : Subsystem  VariantControl=normal_forward_controller
      mask Display:
      | disp('NFC')
      | port_label('input', 1, 'normal in')
      | port_label('input', 2, 'faked in')
      | port_label('output', 1, 'out')
  periodical forward controller : Subsystem  VariantControl=periodical_forward_controller
      mask Display:
      | disp('PFC')
      | port_label('input', 1, 'normal in')
      | port_label('input', 2, 'faked in')
      | port_label('output', 1, 'out')
  step forward controller : Subsystem  VariantControl=step_forward_controller
      mask Display:
      | disp('SFC')
      | port_label('input', 1, 'normal in')
      | port_label('input', 2, 'faked in')
      | port_label('output', 1, 'out')
  output : Outport

== system VACModel/VA Plant/xmv atk block/xmv19 attack controller/Attack Type Controller ==
  note: 1) Only subsystems can be added as variant choices at this level
      | 2) Blocks cannot be connected at this level as connectivity is
      | automatically determined at simulation, based on the active variant
  normal : Inport
  faked : Inport  Port=2
  interval forward controller : Subsystem  VariantControl=interval_forward_controller
      mask Display:
      | disp('IFC')
      | port_label('input', 1, 'normal in')
      | port_label('input', 2, 'faked in')
      | port_label('output', 1, 'out')
  normal forward controller : Subsystem  VariantControl=normal_forward_controller
      mask Display:
      | disp('NFC')
      | port_label('input', 1, 'normal in')
      | port_label('input', 2, 'faked in')
      | port_label('output', 1, 'out')
  periodical forward controller : Subsystem  VariantControl=periodical_forward_controller
      mask Display:
      | disp('PFC')
      | port_label('input', 1, 'normal in')
      | port_label('input', 2, 'faked in')
      | port_label('output', 1, 'out')
  step forward controller : Subsystem  VariantControl=step_forward_controller
      mask Display:
      | disp('SFC')
      | port_label('input', 1, 'normal in')
      | port_label('input', 2, 'faked in')
      | port_label('output', 1, 'out')
  output : Outport

== system VACModel/VA Plant/xmv atk block/xmv2 attack controller/Attack Type Controller ==
  note: 1) Only subsystems can be added as variant choices at this level
      | 2) Blocks cannot be connected at this level as connectivity is
      | automatically determined at simulation, based on the active variant
  normal : Inport
  faked : Inport  Port=2
  interval forward controller : Subsystem  VariantControl=interval_forward_controller
      mask Display:
      | disp('IFC')
      | port_label('input', 1, 'normal in')
      | port_label('input', 2, 'faked in')
      | port_label('output', 1, 'out')
  normal forward controller : Subsystem  VariantControl=normal_forward_controller
      mask Display:
      | disp('NFC')
      | port_label('input', 1, 'normal in')
      | port_label('input', 2, 'faked in')
      | port_label('output', 1, 'out')
  periodical forward controller : Subsystem  VariantControl=periodical_forward_controller
      mask Display:
      | disp('PFC')
      | port_label('input', 1, 'normal in')
      | port_label('input', 2, 'faked in')
      | port_label('output', 1, 'out')
  step forward controller : Subsystem  VariantControl=step_forward_controller
      mask Display:
      | disp('SFC')
      | port_label('input', 1, 'normal in')
      | port_label('input', 2, 'faked in')
      | port_label('output', 1, 'out')
  output : Outport

== system VACModel/VA Plant/xmv atk block/xmv20 attack controller/Attack Type Controller ==
  note: 1) Only subsystems can be added as variant choices at this level
      | 2) Blocks cannot be connected at this level as connectivity is
      | automatically determined at simulation, based on the active variant
  normal : Inport
  faked : Inport  Port=2
  interval forward controller : Subsystem  VariantControl=interval_forward_controller
      mask Display:
      | disp('IFC')
      | port_label('input', 1, 'normal in')
      | port_label('input', 2, 'faked in')
      | port_label('output', 1, 'out')
  normal forward controller : Subsystem  VariantControl=normal_forward_controller
      mask Display:
      | disp('NFC')
      | port_label('input', 1, 'normal in')
      | port_label('input', 2, 'faked in')
      | port_label('output', 1, 'out')
  periodical forward controller : Subsystem  VariantControl=periodical_forward_controller
      mask Display:
      | disp('PFC')
      | port_label('input', 1, 'normal in')
      | port_label('input', 2, 'faked in')
      | port_label('output', 1, 'out')
  step forward controller : Subsystem  VariantControl=step_forward_controller
      mask Display:
      | disp('SFC')
      | port_label('input', 1, 'normal in')
      | port_label('input', 2, 'faked in')
      | port_label('output', 1, 'out')
  output : Outport

== system VACModel/VA Plant/xmv atk block/xmv21 attack controller/Attack Type Controller ==
  note: 1) Only subsystems can be added as variant choices at this level
      | 2) Blocks cannot be connected at this level as connectivity is
      | automatically determined at simulation, based on the active variant
  normal : Inport
  faked : Inport  Port=2
  interval forward controller : Subsystem  VariantControl=interval_forward_controller
      mask Display:
      | disp('IFC')
      | port_label('input', 1, 'normal in')
      | port_label('input', 2, 'faked in')
      | port_label('output', 1, 'out')
  normal forward controller : Subsystem  VariantControl=normal_forward_controller
      mask Display:
      | disp('NFC')
      | port_label('input', 1, 'normal in')
      | port_label('input', 2, 'faked in')
      | port_label('output', 1, 'out')
  periodical forward controller : Subsystem  VariantControl=periodical_forward_controller
      mask Display:
      | disp('PFC')
      | port_label('input', 1, 'normal in')
      | port_label('input', 2, 'faked in')
      | port_label('output', 1, 'out')
  step forward controller : Subsystem  VariantControl=step_forward_controller
      mask Display:
      | disp('SFC')
      | port_label('input', 1, 'normal in')
      | port_label('input', 2, 'faked in')
      | port_label('output', 1, 'out')
  output : Outport

== system VACModel/VA Plant/xmv atk block/xmv22 attack controller/Attack Type Controller ==
  note: 1) Only subsystems can be added as variant choices at this level
      | 2) Blocks cannot be connected at this level as connectivity is
      | automatically determined at simulation, based on the active variant
  normal : Inport
  faked : Inport  Port=2
  interval forward controller : Subsystem  VariantControl=interval_forward_controller
      mask Display:
      | disp('IFC')
      | port_label('input', 1, 'normal in')
      | port_label('input', 2, 'faked in')
      | port_label('output', 1, 'out')
  normal forward controller : Subsystem  VariantControl=normal_forward_controller
      mask Display:
      | disp('NFC')
      | port_label('input', 1, 'normal in')
      | port_label('input', 2, 'faked in')
      | port_label('output', 1, 'out')
  periodical forward controller : Subsystem  VariantControl=periodical_forward_controller
      mask Display:
      | disp('PFC')
      | port_label('input', 1, 'normal in')
      | port_label('input', 2, 'faked in')
      | port_label('output', 1, 'out')
  step forward controller : Subsystem  VariantControl=step_forward_controller
      mask Display:
      | disp('SFC')
      | port_label('input', 1, 'normal in')
      | port_label('input', 2, 'faked in')
      | port_label('output', 1, 'out')
  output : Outport
